simulink model "motor_cc_2"  (R2015a)
settings: Solver=ode45  StartTime=0.0  StopTime=10.0  RelTol=1e-3
undefined symbols (not defined in the file): Bm, J, ka, La, ra
settings Model: Creator=11802972  LastModifiedBy=11802972

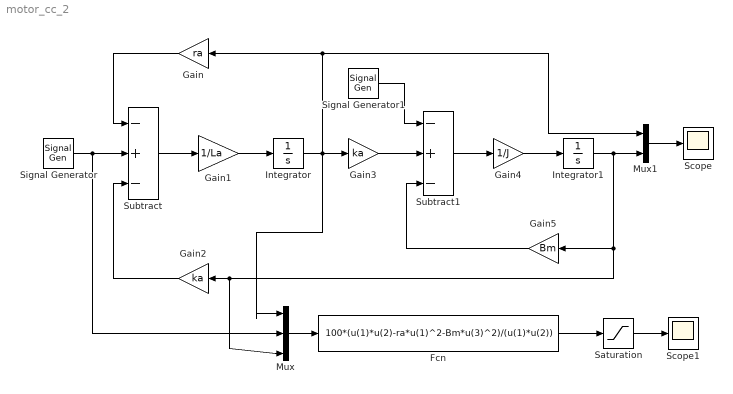
== system motor_cc_2 ==
  Fcn : Fcn  Expr=100*(u(1)*u(2)-ra*u(1)^2-Bm*u(3)^2)/(u(1)*u(2))
  Gain : Gain  Gain=ra
  Gain1 : Gain  Gain=1/La
  Gain2 : Gain  Gain=ka
  Gain3 : Gain  Gain=ka
  Gain4 : Gain  Gain=1/J
  Gain5 : Gain  Gain=Bm
  Integrator : Integrator
  Integrator1 : Integrator
  Mux : Mux  Inputs=3
  Mux1 : Mux  Inputs=2
  Saturation : Saturate  UpperLimit=100  LowerLimit=-100
  Scope : Scope
      settings: TimeRange=10
  Scope1 : Scope
      settings: TimeRange=10
  Signal Generator : SignalGenerator  WaveForm=square  Amplitude=-60  Frequency=2  Units=rad/sec
  Signal Generator1 : SignalGenerator  WaveForm=square  Amplitude=-1  Frequency=2  Units=rad/sec
  Subtract : Sum  Inputs=-+-
  Subtract1 : Sum  Inputs=-+-
  wires:
  Signal Generator/1 -> Mux/2, Subtract/2
  Gain/1 -> Subtract/1
  Subtract/1 -> Gain1/1
  Gain1/1 -> Integrator/1
  Gain2/1 -> Subtract/3
  Integrator/1 -> Mux/1, Mux1/1, Gain/1, Gain3/1
  Gain3/1 -> Subtract1/2
  Signal Generator1/1 -> Subtract1/1
  Subtract1/1 -> Gain4/1
  Gain4/1 -> Integrator1/1
  Gain5/1 -> Subtract1/3
  Integrator1/1 -> Mux1/2, Mux/3, Gain2/1, Gain5/1
  Mux1/1 -> Scope/1
  Mux/1 -> Fcn/1
  Fcn/1 -> Saturation/1
  Saturation/1 -> Scope1/1
